simulink model "energy_aware_controller"  (R2020b)
settings: Solver=VariableStepAuto  StartTime=0.0  StopTime=60  RelTol=1e-3
values from neighbouring files (symbols this model uses):
  b0 = 2 * sqrt(k0 * m_R)    [compliance_PLUS_energy_setup.m]    (also in compliance_adjusting_setup.m = 20; energy_aware_setup.m = 20; optim_criteria.m = 0.2; plot_meshes.m = 0.2)
  E_max = 1    [compliance_PLUS_energy_setup.m]    (also in energy_aware_setup.m = 0.7; optim_criteria.m = 0.5; plot_meshes.m = 0.5; setup.m)
  k0 = 20    [compliance_PLUS_energy_setup.m]    (also in compliance_adjusting_setup.m = 100; energy_aware_setup.m = 100; optim_criteria.m = 1; plot_meshes.m = 1)
  km = 100    [compliance_PLUS_energy_setup.m]    (also in compliance_adjusting_setup.m; energy_aware_setup.m; setup.m)
  m_R = 1    [compliance_PLUS_energy_setup.m]    (also in compliance_adjusting_setup.m; energy_aware_setup.m; setup.m)
  P_max = 1    [compliance_PLUS_energy_setup.m]    (also in energy_aware_setup.m = 0.2; optim_criteria.m = 0.5; plot_meshes.m = 0.5; setup.m = 0.1)
  s0 = 5    [compliance_PLUS_energy_setup.m]    (also in energy_aware_setup.m; setup.m)
  t_collision = 20    [compliance_PLUS_energy_setup.m]    (also in compliance_adjusting_setup.m; energy_aware_setup.m; setup.m)
  t_init = 2    [compliance_PLUS_energy_setup.m]    (also in compliance_adjusting_setup.m; energy_aware_setup.m; setup.m)
  x_O = 0.5    [compliance_PLUS_energy_setup.m]    (also in compliance_adjusting_setup.m; energy_aware_setup.m; setup.m)
  x_R = 0    [compliance_PLUS_energy_setup.m]    (also in compliance_adjusting_setup.m; energy_aware_setup.m; setup.m)
libraries: neural x1
settings Model: Creator=kika  LastModifiedBy=kika

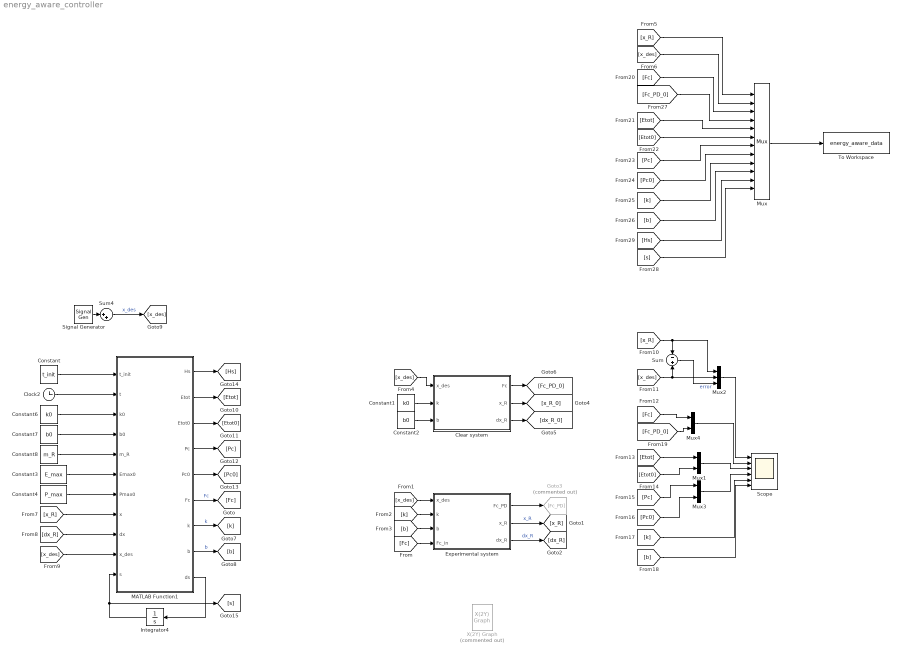
== system energy_aware_controller ==
  Clear system : Subsystem
  Clock2 : Clock
  Constant : Constant  Value=t_init
  Constant1 : Constant  Value=k0
  Constant2 : Constant  Value=b0
  Constant3 : Constant  Value=E_max
  Constant4 : Constant  Value=P_max
  Constant6 : Constant  Value=k0
  Constant7 : Constant  Value=b0
  Constant8 : Constant  Value=m_R
  Experimental system : Subsystem
  Goto3 : Goto  Commented=on  GotoTag=Fc_PD
  Integrator4 : Integrator  InitialCondition=s0
  MATLAB Function1 : MATLAB Function  TreatAsAtomicUnit=on
  Mux : Mux  Inputs=12
  Mux1 : Mux  Inputs=2
  Mux2 : Mux  Inputs=3
  Mux3 : Mux  Inputs=2
  Mux4 : Mux  Inputs=2
  Scope : Scope  NumInputPorts=6
  Signal Generator : SignalGenerator  Frequency=0.5  Units=rad/sec
  Sum : Sum  Inputs=-+
  Sum4 : Sum  Inputs=|++
  To Workspace : ToWorkspace  VariableName=energy_aware_data  SaveFormat=Timeseries  SampleTime=-1
  X(2Y) Graph : neural/Control Systems/X(2Y)  Graph  Commented=on  xmin=0  xmax=5  ymin=21  ymax=22  st=-1
      settings: SourceProductBaseCode=NN
  wires:
  Constant4/1 -> MATLAB Function1/7(Pmax0)
  Constant3/1 -> MATLAB Function1/6(Emax0)
  MATLAB Function1/9(ds) -> Integrator4/1
  Constant7/1 -> MATLAB Function1/4(b0)
  MATLAB Function1/7(k) -> [k]  "k"
  Constant8/1 -> MATLAB Function1/5(m_R)
  Constant6/1 -> MATLAB Function1/3(k0)
  Integrator4/1 -> MATLAB Function1/11(s), [s]
  Clock2/1 -> MATLAB Function1/2(t)
  MATLAB Function1/8(b) -> [b]  "b"
  Signal Generator/1 -> Sum4/1
  Constant/1 -> MATLAB Function1/1(t_init)
  MATLAB Function1/6(Fc) -> [Fc]  "Fc"
  [Fc] -> Experimental system/4(Fc_in)
  [x_des] -> Experimental system/1(x_des)
  Experimental system/2(x_R) -> [x_R]  "x_R"
  Experimental system/3(dx_R) -> [dx_R]  "dx_R"
  Experimental system/1(Fc_PD) -> Goto3/1
  Clear system/1(Fc) -> [Fc_PD_0]
  Clear system/2(x_R) -> [x_R_0]
  Clear system/3(dx_R) -> [dx_R_0]
  [k] -> Experimental system/2(k)
  [b] -> Experimental system/3(b)
  [x_des] -> Clear system/1(x_des)
  Constant1/1 -> Clear system/2(k)
  Constant2/1 -> Clear system/3(b)
  [dx_R] -> MATLAB Function1/9(dx)
  [x_R] -> MATLAB Function1/8(x)
  Sum4/1 -> [x_des]  "x_des"
  [x_des] -> MATLAB Function1/10(x_des)
  [x_R] -> Sum/1, Mux2/1
  [x_des] -> Mux2/2, Sum/2
  Mux2/1 -> Scope/1
  [Fc] -> Mux4/1
  MATLAB Function1/5(Pc0) -> [Pc0]
  MATLAB Function1/4(Pc) -> [Pc]
  MATLAB Function1/3(Etot0) -> [Etot0]
  MATLAB Function1/2(Etot) -> [Etot]
  MATLAB Function1/1(Hs) -> [Hs]
  [Etot] -> Mux1/1
  [Etot0] -> Mux1/2
  [Pc0] -> Mux3/2
  [Pc] -> Mux3/1
  Mux1/1 -> Scope/3
  Mux3/1 -> Scope/4
  [k] -> Scope/5
  [b] -> Scope/6
  [Fc_PD_0] -> Mux4/2
  Mux4/1 -> Scope/2
  Sum/1 -> Mux2/3  "error"
  [Fc_PD_0] -> Mux/4
  [Fc] -> Mux/3
  [Etot] -> Mux/5
  [Etot0] -> Mux/6
  [x_des] -> Mux/2
  [x_R] -> Mux/1
  [Pc] -> Mux/7
  [Pc0] -> Mux/8
  [k] -> Mux/9
  [b] -> Mux/10
  Mux/1 -> To Workspace/1
  [Hs] -> Mux/11
  [s] -> Mux/12

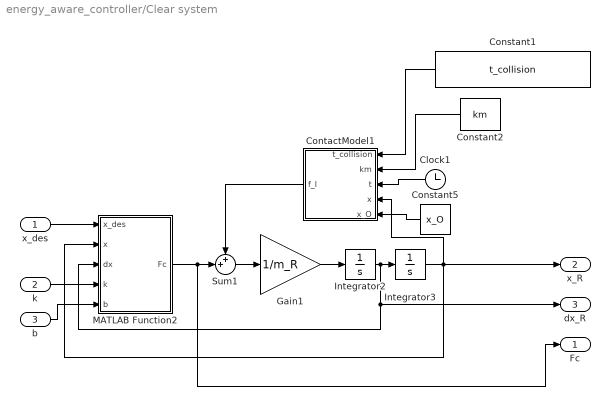
== system energy_aware_controller/Clear system ==
  x_des : Inport
  k : Inport  Port=2
  b : Inport  Port=3
  Clock1 : Clock
  Constant1 : Constant  Value=t_collision
  Constant2 : Constant  Value=km
  Constant5 : Constant  Value=x_O
  ContactModel1 : MATLAB Function  TreatAsAtomicUnit=on
  Gain1 : Gain  Gain=1/m_R
  Integrator2 : Integrator
  Integrator3 : Integrator  InitialCondition=x_R
  MATLAB Function2 : MATLAB Function  TreatAsAtomicUnit=on
  Sum1 : Sum  Inputs=++|
  Fc : Outport
  x_R : Outport  Port=2
  dx_R : Outport  Port=3
  wires:
  k/1 -> MATLAB Function2/4(k)
  ContactModel1/1(f_I) -> Sum1/1
  Clock1/1 -> ContactModel1/3(t)
  Integrator3/1 -> x_R/1, ContactModel1/4(x), MATLAB Function2/2(x)
  x_des/1 -> MATLAB Function2/1(x_des)
  b/1 -> MATLAB Function2/5(b)
  Sum1/1 -> Gain1/1
  Constant5/1 -> ContactModel1/5(x_O)
  Gain1/1 -> Integrator2/1
  MATLAB Function2/1(Fc) -> Fc/1, Sum1/2
  Integrator2/1 -> dx_R/1, MATLAB Function2/3(dx), Integrator3/1
  Constant1/1 -> ContactModel1/1(t_collision)
  Constant2/1 -> ContactModel1/2(km)

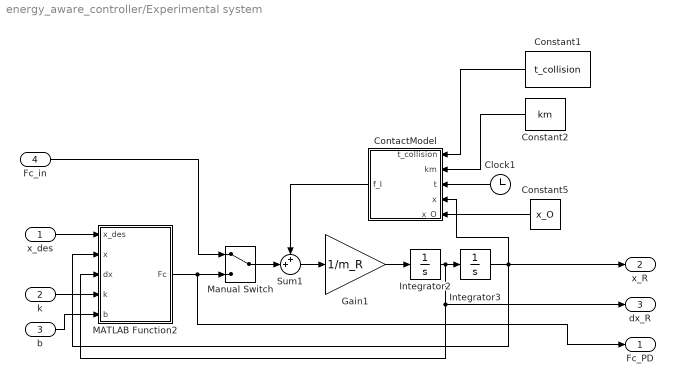
== system energy_aware_controller/Experimental system ==
  x_des : Inport
  k : Inport  Port=2
  b : Inport  Port=3
  Fc_in : Inport  Port=4
  Clock1 : Clock
  Constant1 : Constant  Value=t_collision
  Constant2 : Constant  Value=km
  Constant5 : Constant  Value=x_O
  ContactModel : MATLAB Function  TreatAsAtomicUnit=on
  Gain1 : Gain  Gain=1/m_R
  Integrator2 : Integrator
  Integrator3 : Integrator  InitialCondition=x_R
  MATLAB Function2 : MATLAB Function  TreatAsAtomicUnit=on
  Manual Switch : ManualSwitch
  Sum1 : Sum  Inputs=++|
  Fc_PD : Outport
  x_R : Outport  Port=2
  dx_R : Outport  Port=3
  wires:
  k/1 -> MATLAB Function2/4(k)
  ContactModel/1(f_I) -> Sum1/1
  Clock1/1 -> ContactModel/3(t)
  Integrator3/1 -> x_R/1, ContactModel/4(x), MATLAB Function2/2(x)
  x_des/1 -> MATLAB Function2/1(x_des)
  b/1 -> MATLAB Function2/5(b)
  Sum1/1 -> Gain1/1
  Constant5/1 -> ContactModel/5(x_O)
  Gain1/1 -> Integrator2/1
  MATLAB Function2/1(Fc) -> Manual Switch/2, Fc_PD/1
  Integrator2/1 -> dx_R/1, MATLAB Function2/3(dx), Integrator3/1
  Constant1/1 -> ContactModel/1(t_collision)
  Constant2/1 -> ContactModel/2(km)
  Fc_in/1 -> Manual Switch/1
  Manual Switch/1 -> Sum1/2

== matlab function energy_aware_controller/Experimental system/ContactModel ==
  data: t_collision input; km input; t input; f_I output; x input; x_O input
function f_I = fcn(t_collision, km, t, x, x_O)


f_I = 0;

if t > t_collision
    if x > x_O
        f_I = km * (x_O - x);
    end
end

== matlab function energy_aware_controller/Experimental system/MATLAB Function2 ==
  data: x_des input; Fc output; x input; dx input; k input; b input
function Fc = fcn(x_des, x, dx, k, b)

Fc = k * (x_des - x) - b * dx;

== matlab function energy_aware_controller/MATLAB Function1 ==
  data: t_init input; t input; k0 input; b0 input; m_R input; Hs output; Emax0 input; Pmax0 input; Etot output; Etot0 output; Pc output; Pc0 output; Fc output; x input; k output; b output; dx input; x_des input; s input; ds output
function [Hs, Etot, Etot0, Pc, Pc0, Fc, k, b, ds] = energy_aware(t_init,t, k0, b0, m_R, Emax0, Pmax0, x, dx, x_des, s)
    
    % initialisation time
    Emax = 1000;
    Pmax = 2000;
    if t > t_init
        Emax = Emax0;
        Pmax = Pmax0;
    end

    e = x_des - x;  % control error
    
    % Kinetic energy
    T = 0.5 * m_R * dx^2;

    % stiffness abjusting using initial Potential energy
    V0 = 0.5 * k0 * e^2;
    Etot0 = T + V0;
    k = k0;
    if Etot0 > Emax
        k = (Emax - T) / (0.5 * e^2);
    end

    % damping adjusting using new stiffness
    Fs = k * e;
    Fd0 = b0 * dx;
    Fc0 = Fs - Fd0;
    Pc0 = Fc0 * dx;
    b = b0;
    if Pc0 > Pmax
        b = (Fs * dx - Pmax) / dx^2;
    end

    % new control
    Fd = b * dx;
    Fc = Fs - Fd; % control without passivity

    % adjusted total Energy and Power
    V = 0.5 * k * e^2;
    Etot = T + V;
    Pc = Fc * dx;

    % Passivity
    eps = 0.1;
    Hs = 0.5 * s^2;

    u = -Fc * s / sqrt(2 * eps);    % or u = 0;
    if Hs >= eps || Pc < 0
        u = - Fc / s;
    end

    % total contol with passivity
    Fc = -u * s;
    ds = u * dx;

== matlab function energy_aware_controller/Clear system/MATLAB Function2 ==
  data: x_des input; Fc output; x input; dx input; k input; b input
function Fc = fcn(x_des, x, dx, k, b)

Fc = k * (x_des - x) - b * dx;

== matlab function energy_aware_controller/Clear system/ContactModel1 ==
  data: t_collision input; km input; t input; f_I output; x input; x_O input
function f_I = fcn(t_collision, km, t, x, x_O)


f_I = 0;

if t > t_collision
    if x > x_O
        f_I = km * (x_O - x);
    end
end
